simulink model "physics_model"  (R2026a)
settings: Solver=VariableStepAuto
values from neighbouring files (symbols this model uses):
  params = base    [build_params.m]    (also in run_initial.m = rig())
settings Model: Creator=hardik-karan  LastModifiedBy=hardik-karan

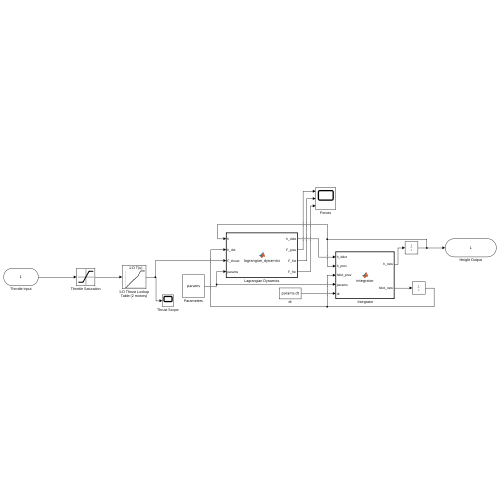
[thumbnail: Simulink's stored preview of the top-level diagram]
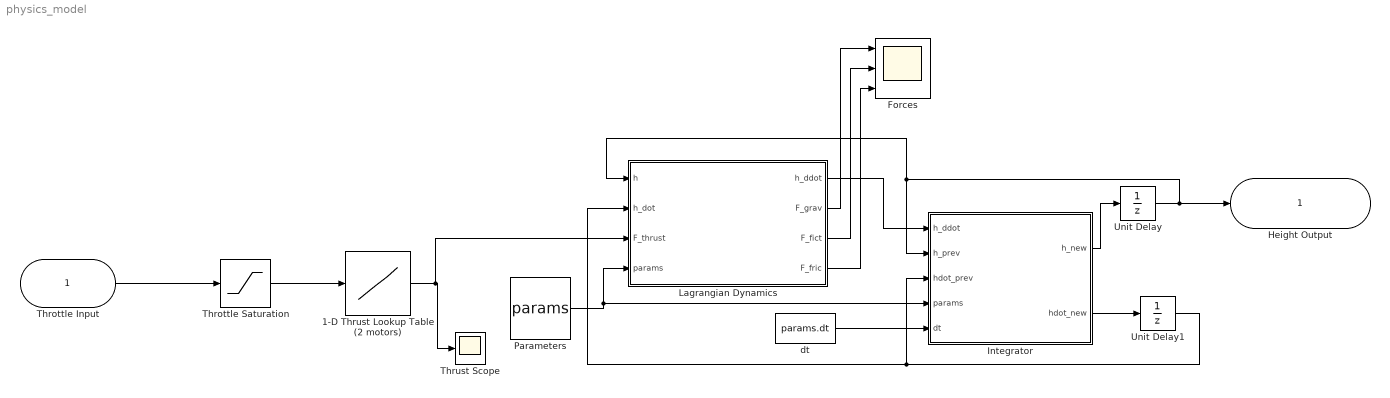
== system physics_model ==
  Throttle Input : Inport
  " Integrator" : MATLAB Function  TreatAsAtomicUnit=on
  1-D Thrust Lookup Table (2 motors) : Lookup_n-D  NumberOfTableDimensions=1  BreakpointsForDimension1=params.throttle_grid  Table=params.thrust_grid  ExtrapMethod=Clip  InternalRulePriority=Speed  RndMeth=Simplest
  Forces : Scope  NumInputPorts=3
  Lagrangian Dynamics : MATLAB Function  TreatAsAtomicUnit=on
  Parameters : Constant  Value=params
  Throttle Saturation : Saturate  UpperLimit=80  LowerLimit=0
  Thrust Scope : Scope
      settings: ActiveDisplayYMinimum=9.6502299000333984  ActiveDisplayYMaximum=22.916190651115247
  Unit Delay : UnitDelay  SampleTime=-1
  Unit Delay1 : UnitDelay  SampleTime=-1
  dt : Constant  Value=params.dt
  Height Output : Outport
  wires:
  Throttle Saturation/1 -> 1-D Thrust Lookup Table (2 motors)/1
  Throttle Input/1 -> Throttle Saturation/1
  1-D Thrust Lookup Table (2 motors)/1 -> Lagrangian Dynamics/3(F_thrust), Thrust Scope/1
  Parameters/1 -> Lagrangian Dynamics/4(params), " Integrator"/4(params)
  Lagrangian Dynamics/1(h_ddot) -> " Integrator"/1(h_ddot)
  dt/1 -> " Integrator"/5(dt)
  " Integrator"/1(h_new) -> Unit Delay/1
  Unit Delay/1 -> Height Output/1, " Integrator"/2(h_prev), Lagrangian Dynamics/1(h)
  " Integrator"/2(hdot_new) -> Unit Delay1/1
  Unit Delay1/1 -> " Integrator"/3(hdot_prev), Lagrangian Dynamics/2(h_dot)
  Lagrangian Dynamics/2(F_grav) -> Forces/1
  Lagrangian Dynamics/3(F_fict) -> Forces/2
  Lagrangian Dynamics/4(F_fric) -> Forces/3

== matlab function physics_model/ Integrator ==
  data: h_ddot input; h_new output; h_prev input; hdot_prev input; params input; dt input; hdot_new output
function [h_new, hdot_new] = integrator(h_ddot, h_prev, hdot_prev, params, dt)
    hdot_new = hdot_prev + h_ddot * dt;
    h_new = h_prev + hdot_new * dt;
    if h_new >= params.h_max && hdot_new > 0
        h_new = params.h_max; hdot_new = 0;
    elseif h_new <= params.h_min && hdot_new < 0
        h_new = params.h_min; hdot_new = 0;
    end
end

== matlab function physics_model/Lagrangian Dynamics ==
  data: h input; h_ddot output; h_dot input; F_thrust input; params input; F_grav output; F_fict output; F_fric output
function [h_ddot, F_grav, F_fict, F_fric] = lagrangian_dynamics(h, h_dot, F_thrust, params)
    [h_ddot, F_grav, F_fict, F_fric] = lagrangian(h, h_dot, F_thrust, params);
end
